simulink model "GenerateQuartenionBus"  (R2017a)
settings: Solver=FixedStepAuto  StartTime=0.0  StopTime=20  FixedStep=0.05  RelTol=1e-3  EnableMultiTasking=on
PreLoadFcn:
  | myBusDef
StartFcn:
  | % Full path to the block
  | blk = 'GenerateQuartenionBus/Bus Creator';
  | 
  | % Attach the event listener
  | h = add_exec_event_listener(blk, ...
  |          'PostOutputs', @RTVisualisation);
settings Model: Creator=felip  LastModifiedBy=felip

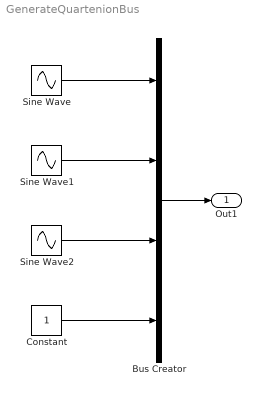
== system GenerateQuartenionBus ==
  Bus Creator : BusCreator  Inputs=4  OutDataTypeStr=Bus: BO  NonVirtualBus=on
  Constant : Constant
  Sine Wave : Sin  Phase=pi/2  SampleTime=0
  Sine Wave1 : Sin  Amplitude=0.5  SampleTime=0
  Sine Wave2 : Sin  Amplitude=0.5  Phase=pi/4  SampleTime=0
  Out1 : Outport
  wires:
  Sine Wave1/1 -> Bus Creator/2
  Sine Wave/1 -> Bus Creator/1
  Bus Creator/1 -> Out1/1
  Constant/1 -> Bus Creator/4
  Sine Wave2/1 -> Bus Creator/3
